simulink model "phase4_lab_full_students"  (R2023b)
settings: Solver=ode4  StartTime=0.0  StopTime=inf  FixedStep=Ts  RelTol=1e-3  EnableMultiTasking=on
values from neighbouring files (symbols this model uses):
  A = [zeros(2,2)  eye(2) ... (first row only)    [Task2_P4.m]    (also in linearized_model_students.m; task1_P4.m; task1_p4.m; task2_P4.m)
  B = [zeros(2,1) ... (first row only)    [Task2_P4.m]    (also in linearized_model_students.m; task1_P4.m; task1_p4.m; task2_P4.m)
  C = [1 0 0 0 ... (first row only)    [Task2_P4.m]    (also in linearized_model_students.m; task1_P4.m; task1_p4.m; task2_P4.m)
  Kf = Kc * T_1    [Task2_P4.m]    (also in linearized_model_students.m; task1_P4.m; task1_p4.m; task2_P4.m)
  L = Lt.'    [Task3_p4.m]    (also in linearized_model_students.m; task3_P4.m)
  q20 = pi    (= 3.14159265359)    [Task2_P4.m]    (also in linearized_model_students.m; task1_P4.m; task1_p4.m; task2_P4.m)
undefined symbols (not defined in the file or in its folder): HIL, qc_get_step_size
libraries: simulink x3, quarc_library x3
settings Model: SimulationMode=external  ExtModeTrigDuration=40000  Creator=MLevis  LastModifiedBy=smitj19
settings SolverCC: AlgebraicLoopSolver=TrustRegion  PositivePriorityOrder=on
settings DataIOCC: LimitDataPoints=on  SaveFormat=Array  SignalLoggingSaveFormat=ModelDataLogs
settings OptimizationCC: ReuseModelBlockBuffer=off  ExpressionDepthLimit=2147483647
settings DebuggingCC: UnderspecifiedInitializationDetection=Classic  MergeDetectMultiDrivingBlocksExec=none  SolverPrmCheckMsg=warning  FcnCallInpInsideContextMsg=warning  UnconnectedInputMsg=warning  UnconnectedOutputMsg=warning  UnconnectedLineMsg=warning  StateNameClashWarn=warning  SFUnexpectedBacktrackingDiag=warning  SFNoUnconditionalDefaultTransitionDiag=warning  SFExecutionAtInitializationDiag=none  ArithmeticOperatorsInVariantConditions=warning
settings ModelReferenceCC: EnableRefExpFcnMdlSchedulingChecks=on  PropagateSignalLabelsOutOfModel=off
settings SFSimCC: SimUseLocalCustomCode=off  CustomCodeUndefinedFunction=UseInterfaceOnly
settings RTWCC: Description=QUARC Win64 Target Using Toolchain  SystemTargetFile=quarc_win64.tlc  TemplateMakefile=quarc_default_tmf  RTWUseLocalCustomCode=off  Toolchain=QUARC win64 | nmake (64-bit Windows)  BuildConfiguration=Faster Runs
settings CodeAppCC: StateflowObjectComments=on
settings STFCustomTargetCC: TargetLangStandard=C89/C90 (ANSI)  ConcurrentExecutionCompliant=on  GRTInterface=on  UseToolchainInfoCompliant=on  SystemTargetFile=quarc_win64.tlc
settings GRTTargetCC: TargetLangStandard=C89/C90 (ANSI)  ParMdlRefBuildCompliant=off  CompOptLevelCompliant=off  CombineOutputUpdateFcns=off  MatFileLogging=off  CPPClassGenCompliant=off  GRTInterface=on  ExtMode=on  ExtModeMexFile=quarc_comm
settings ConfigComp: CovMetricSettings=dw  CovSaveCumulativeToWorkspaceVar=on  CovSaveSingleToWorkspaceVar=on  CovExternalEMLEnable=off  CovSFcnEnable=off

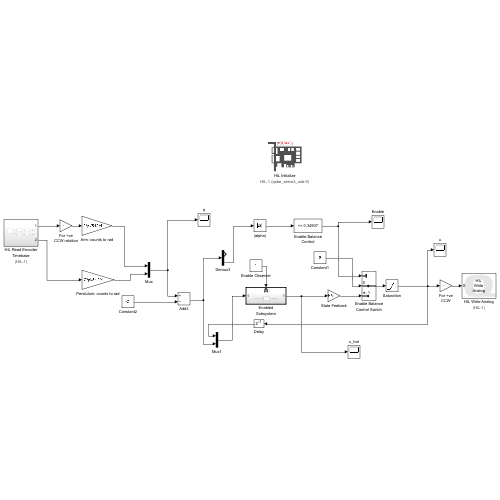
[thumbnail: Simulink's stored preview of the top-level diagram]
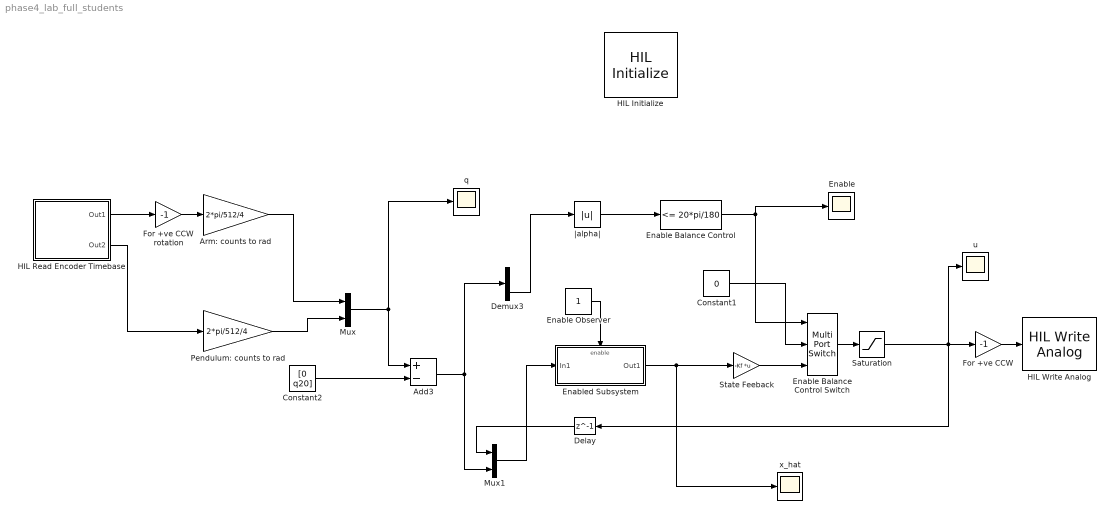
== system phase4_lab_full_students ==
  Add3 : Sum  Inputs=+-
  Arm: counts to rad : Gain  Gain=2*pi/512/4
  Constant1 : Constant  Value=0
  Constant2 : Constant  Value="[0  q20]"
  Delay : Delay  DelayLength=1  InitialCondition=0
  Demux3 : Demux  Outputs=2
  Enable : Scope
  Enable Balance Control : simulink/Logic and Bit Operations/Compare To Constant  relop=<=  const=20*pi/180  OutDataTypeStr=uint8  ZeroCross=off
  Enable Balance Control Switch : MultiPortSwitch  DataPortOrder=Zero-based contiguous  Inputs=2  zeroidx=on  SaturateOnIntegerOverflow=off  InputSameDT=off
  Enable Observer : Constant
  Enabled Subsystem : Subsystem  TreatAsAtomicUnit=on
  For +ve CCW : Gain  Gain=-1
  For +ve CCW rotation : Gain  Gain=-1
  HIL Initialize : quarc_library/Data Acquisition/Generic/Configuration/HIL Initialize  object_name=HIL-1  board_type=qube_servo3_usb  board_number=0  board_options=pwm_en=0  exclusive=off  active=off  hardware_clocks=[0]  clock_modes=[]  initial_clock_frequencies=[]  set_clock_params_at_start=off  set_clock_params_at_switch_in=off  set_clock_frequencies_at_start=off  set_clock_frequencies_at_switch_in=off  analog_input_channels=[0]  analog_input_configurations=[]  analog_input_maximums=3  analog_input_minimums=-3  set_analog_input_params_at_start=off  set_analog_input_params_at_switch_in=off  analog_output_channels=[0]  analog_output_maximums=15  analog_output_minimums=-15  initial_analog_outputs=[0]  final_analog_outputs=[0]  watchdog_analog_outputs=0  set_analog_output_params_at_start=off  set_analog_output_params_at_switch_in=off  set_analog_outputs_at_start=on  set_analog_outputs_at_switch_in=off  set_analog_outputs_at_terminate=on  set_analog_outputs_at_switch_out=off  set_analog_outputs_on_watchdog=on  digital_input_channels=[]  digital_output_channels=[0]  digital_output_configuration=[]  initial_digital_outputs=[1]  final_digital_outputs=[0]  watchdog_digital_outputs=[0]  set_digital_output_params_at_start=off  set_digital_output_params_at_switch_in=off  set_digital_outputs_at_start=on  set_digital_outputs_at_switch_in=off  set_digital_outputs_at_terminate=on  set_digital_outputs_at_switch_out=off  set_digital_outputs_on_watchdog=on  encoder_channels=[0:1]  quadrature=[4]  encoder_filter_frequency=[]  initial_encoder_counts=[0]  set_encoder_params_at_start=off  set_encoder_params_at_switch_in=off  set_encoder_counts_at_start=on  set_encoder_counts_at_switch_in=off  pwm_channels=[]  pwm_modes=[0]  pwm_frequency=23195  pwm_configuration=[1]  pwm_alignment=[0]  pwm_polarity=[1]  pwm_leading_deadband=[0]  pwm_trailing_deadband=[0]  initial_pwm_outputs=[0]  final_pwm_outputs=[0]  watchdog_pwm_outputs=[]  set_pwm_params_at_start=off  set_pwm_params_at_switch_in=off  set_pwm_outputs_at_start=off  set_pwm_outputs_at_switch_in=off  set_pwm_outputs_at_terminate=off  set_pwm_outputs_at_switch_out=off  set_pwm_outputs_on_watchdog=off  other_output_channels=[11000:11002]  initial_other_outputs=[0 1 0]  final_other_outputs=[1 0 0]  watchdog_other_outputs=[0 0 1]  set_other_outputs_at_start=on  set_other_outputs_at_switch_in=off  set_other_outputs_at_terminate=on  set_other_outputs_at_switch_out=off  set_other_outputs_on_watchdog=on
  HIL Read Encoder Timebase : Subsystem  Tag=(HIL-1)  Description=Qube-Servo 3 encoder glitch workaround
      settings: AttributesFormatString=%<Tag>
  HIL Write Analog : quarc_library/Data Acquisition/Generic/Immediate I//O/HIL Write Analog  object_name=HIL-1  channels=0  sample_time=-1  active=off  vector_input=off
  Mux : Mux  Inputs=2
  Mux1 : Mux  Inputs=2
  Pendulum: counts to rad : Gain  Gain=2*pi/512/4
  Saturation : Saturate  UpperLimit=5  LowerLimit=-5
  State Feeback : Gain  Gain=-Kf  Multiplication=Matrix(K*u)
  q : Scope
  u : Scope
  x_hat : Scope
  |alpha| : Abs  SaturateOnIntegerOverflow=off
  wires:
  For +ve CCW/1 -> HIL Write Analog/1
  For +ve CCW rotation/1 -> Arm: counts to rad/1
  Arm: counts to rad/1 -> Mux/1
  Mux/1 -> Add3/1, q/1
  Pendulum: counts to rad/1 -> Mux/2
  Enable Balance Control Switch/1 -> Saturation/1
  HIL Read Encoder Timebase/1(Out1) -> For +ve CCW rotation/1
  HIL Read Encoder Timebase/2(Out2) -> Pendulum: counts to rad/1
  Constant2/1 -> Add3/2
  Demux3/2 -> |alpha|/1
  Add3/1 -> Mux1/2, Demux3/1
  State Feeback/1 -> Enable Balance Control Switch/3
  Constant1/1 -> Enable Balance Control Switch/2
  |alpha|/1 -> Enable Balance Control/1
  Enabled Subsystem/1(Out1) -> x_hat/1, State Feeback/1
  Mux1/1 -> Enabled Subsystem/1(In1)
  Enable Balance Control/1 -> Enable Balance Control Switch/1, Enable/1
  Delay/1 -> Mux1/1
  Saturation/1 -> u/1, Delay/1, For +ve CCW/1
  Enable Observer/1 -> Enabled Subsystem/Enable

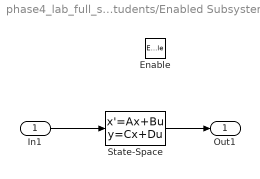
== system phase4_lab_full_students/Enabled Subsystem ==
  In1 : Inport
  Enable : EnablePort
  State-Space : StateSpace  A=A-L*C  B=[B L]  C=eye(4)  D=zeros(4,3)  InitialCondition=[0;0;0;0]
  Out1 : Outport
  wires:
  State-Space/1 -> Out1/1
  In1/1 -> State-Space/1

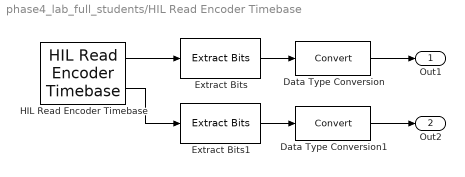
== system phase4_lab_full_students/HIL Read Encoder Timebase ==
  Data Type Conversion : DataTypeConversion  SaturateOnIntegerOverflow=off  RndMeth=Floor
  Data Type Conversion1 : DataTypeConversion  SaturateOnIntegerOverflow=off  RndMeth=Floor
  Extract Bits : simulink/Logic and Bit Operations/Extract Bits  bitsToExtract=Lower half  numBits=16  bitIdxRange=[0 7]  outScalingMode=Preserve fixed-point scaling
  Extract Bits1 : simulink/Logic and Bit Operations/Extract Bits  bitsToExtract=Lower half  numBits=16  bitIdxRange=[0 7]  outScalingMode=Preserve fixed-point scaling
  HIL Read Encoder Timebase : quarc_library/Data Acquisition/Generic/Timebases/HIL Read Encoder Timebase  object_name=HIL-1  clock=0  channels=[0:1]  active=on  vector_output=off  data_type_mode=Specify via dialog  data_type=int32  overflow_mode=Error on overflow  samples_in_buffer=max(ceil(1/qc_get_step_size), 1)
  Out1 : Outport
  Out2 : Outport  Port=2
  wires:
  HIL Read Encoder Timebase/1 -> Extract Bits/1
  HIL Read Encoder Timebase/2 -> Extract Bits1/1
  Extract Bits/1 -> Data Type Conversion/1
  Extract Bits1/1 -> Data Type Conversion1/1
  Data Type Conversion/1 -> Out1/1
  Data Type Conversion1/1 -> Out2/1
